simulink model "value_out_of_bounds"  (R2017a)
settings: Solver=VariableStepAuto  StartTime=0.0  StopTime=10.0  RelTol=1e-3
settings Model: Creator=joaomanito  LastModifiedBy=joaomanito

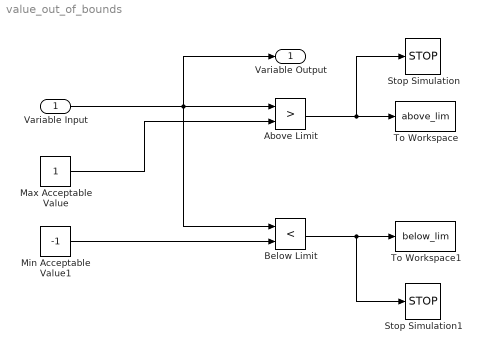
== system value_out_of_bounds ==
  Variable Input : Inport
  Above Limit : RelationalOperator  Operator=>  OutDataTypeStr=boolean  RndMeth=Simplest
  Below Limit : RelationalOperator  Operator=<  OutDataTypeStr=boolean  RndMeth=Simplest
  Max Acceptable Value : Constant
  Min Acceptable Value1 : Constant  Value=-1
  Stop Simulation : Stop
  Stop Simulation1 : Stop
  To Workspace : ToWorkspace  VariableName=above_lim  SaveFormat=Timeseries  SampleTime=-1
      settings: MaxDataPoints=1
  To Workspace1 : ToWorkspace  VariableName=below_lim  SaveFormat=Timeseries  SampleTime=-1
  Variable Output : Outport
  wires:
  Variable Input/1 -> Variable Output/1, Below Limit/1, Above Limit/1
  Max Acceptable Value/1 -> Above Limit/2
  Min Acceptable Value1/1 -> Below Limit/2
  Below Limit/1 -> Stop Simulation1/1, To Workspace1/1
  Above Limit/1 -> Stop Simulation/1, To Workspace/1
